simulink model "controladores_con_modulador"  (R2023b)
settings: Solver=FixedStepAuto  StartTime=0.0  StopTime=10.0  RelTol=1e-3
undefined symbols (not defined in the file): bh_eq_prima, DiscIntNeverNeededParam, i_h, Jh_eq_aux, Kd_h, Kd_t, Ki_h, Ki_t, Kp_h, Kp_t, r_hd, T_hm_max, T_s2, T_tm_max, tau_hm, tau_tm
settings Model: Creator=Ferran  LastModifiedBy=Ferran

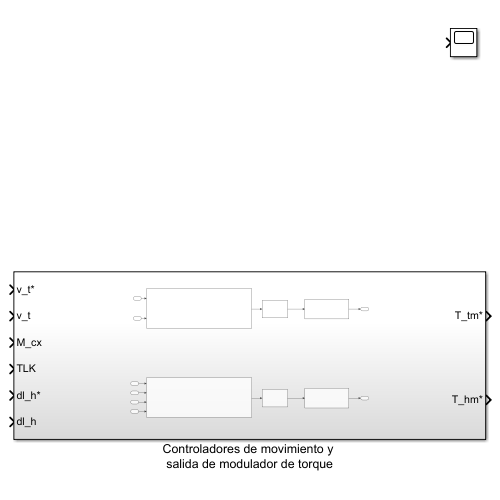
[thumbnail: Simulink's stored preview of the top-level diagram]
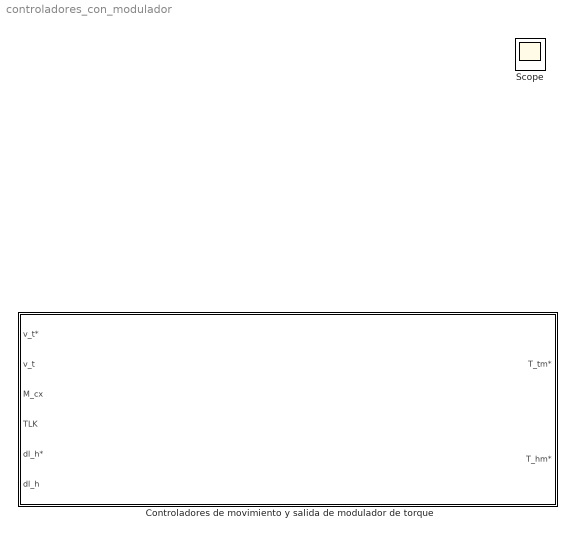
== system controladores_con_modulador ==
  Controladores de movimiento y salida de modulador de torque : Subsystem
  Scope : Scope

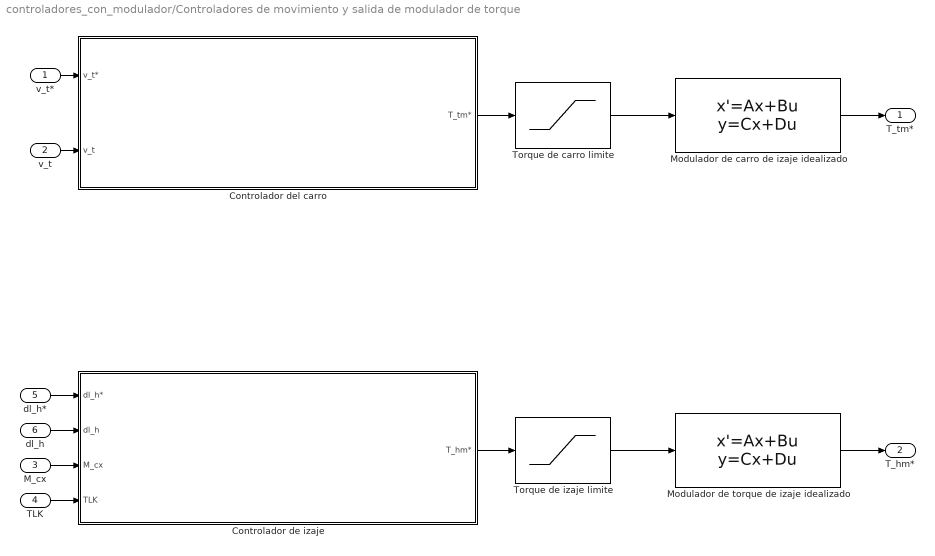
== system controladores_con_modulador/Controladores de movimiento y salida de modulador de torque ==
  v_t* : Inport
  v_t : Inport  Port=2
  M_cx : Inport  Port=3
  TLK : Inport  Port=4
  dl_h* : Inport  Port=5
  dl_h : Inport  Port=6
  Controlador de izaje : Subsystem
  Controlador del carro : Subsystem
  Modulador de carro de izaje idealizado : StateSpace  A=-1/tau_tm  B=1/tau_tm  D=0  InitialCondition=0
  Modulador de torque de izaje idealizado : StateSpace  A=-1/tau_hm  B=1/tau_hm  D=0  InitialCondition=0
  Torque de carro limite : Saturate  UpperLimit=T_tm_max  LowerLimit=-T_tm_max
  Torque de izaje limite : Saturate  UpperLimit=T_hm_max  LowerLimit=-T_hm_max
  T_tm* : Outport
  T_hm* : Outport  Port=2
  wires:
  dl_h*/1 -> Controlador de izaje/1(dl_h*)
  v_t/1 -> Controlador del carro/2(v_t)
  v_t*/1 -> Controlador del carro/1(v_t*)
  Controlador de izaje/1(T_hm*) -> Torque de izaje limite/1
  Controlador del carro/1(T_tm*) -> Torque de carro limite/1
  TLK/1 -> Controlador de izaje/4(TLK)
  dl_h/1 -> Controlador de izaje/2(dl_h)
  M_cx/1 -> Controlador de izaje/3(M_cx)
  Torque de izaje limite/1 -> Modulador de torque de izaje idealizado/1
  Torque de carro limite/1 -> Modulador de carro de izaje idealizado/1
  Modulador de carro de izaje idealizado/1 -> T_tm*/1
  Modulador de torque de izaje idealizado/1 -> T_hm*/1

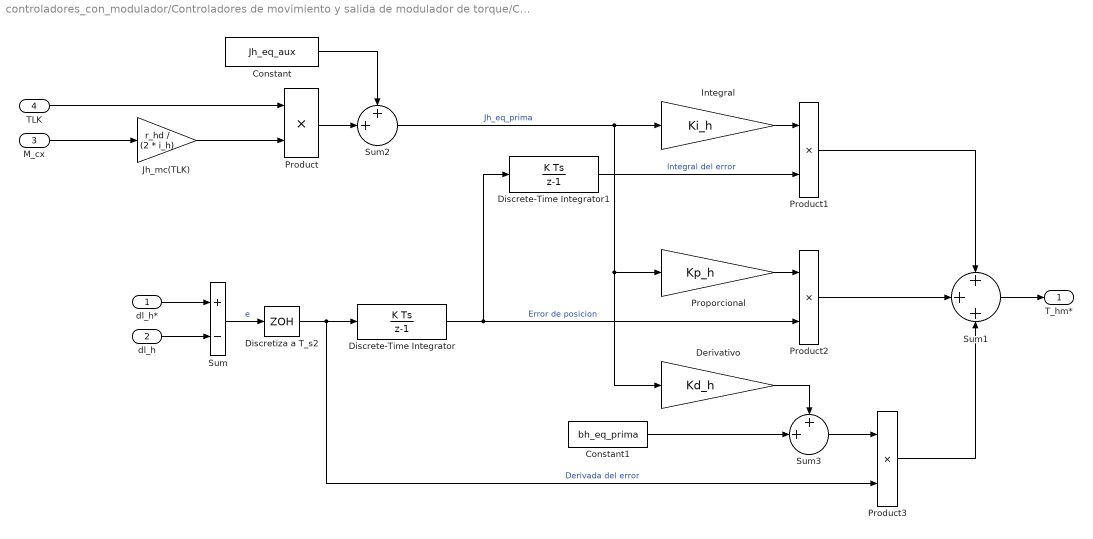
== system controladores_con_modulador/Controladores de movimiento y salida de modulador de torque/Controlador de izaje ==
  dl_h* : Inport
  dl_h : Inport  Port=2
  M_cx : Inport  Port=3
  TLK : Inport  Port=4
  Constant : Constant  Value=Jh_eq_aux
  Constant1 : Constant  Value=bh_eq_prima
  Derivativo : Gain  Gain=Kd_h
  Discrete-Time Integrator : DiscreteIntegrator  SampleTime=T_s2  ICPrevOutput=DiscIntNeverNeededParam  ICPrevScaledInput=DiscIntNeverNeededParam
  Discrete-Time Integrator1 : DiscreteIntegrator  SampleTime=T_s2  ICPrevOutput=DiscIntNeverNeededParam  ICPrevScaledInput=DiscIntNeverNeededParam
  Discretiza a T_s2 : ZeroOrderHold  SampleTime=T_s2
  Integral : Gain  Gain=Ki_h
  Jh_mc(TLK) : Gain  Gain=r_hd / (2 * i_h)
  Product{,1..3} (4 alike) : Product
  Proporcional : Gain  Gain=Kp_h
  Sum : Sum  Inputs=+-
  Sum1 : Sum  Inputs=+++
  Sum2 : Sum  Inputs=++|
  Sum3 : Sum  Inputs=++|
  T_hm* : Outport
  wires:
  dl_h*/1 -> Sum/1
  Product1/1 -> Sum1/1
  Discretiza a T_s2/1 -> Discrete-Time Integrator/1, Product3/2  "Derivada del error"
  dl_h/1 -> Sum/2
  Product3/1 -> Sum1/3
  Sum1/1 -> T_hm*/1
  Sum/1 -> Discretiza a T_s2/1  "e"
  Discrete-Time Integrator1/1 -> Product1/2  "Integral del error"
  M_cx/1 -> Jh_mc(TLK)/1
  Jh_mc(TLK)/1 -> Product/2
  TLK/1 -> Product/1
  Product/1 -> Sum2/2
  Constant/1 -> Sum2/1
  Sum2/1 -> Derivativo/1, Proporcional/1, Integral/1  "Jh_eq_prima"
  Integral/1 -> Product1/1
  Proporcional/1 -> Product2/1
  Discrete-Time Integrator/1 -> Product2/2, Discrete-Time Integrator1/1  "Error de posicion"
  Product2/1 -> Sum1/2
  Constant1/1 -> Sum3/2
  Derivativo/1 -> Sum3/1
  Sum3/1 -> Product3/1

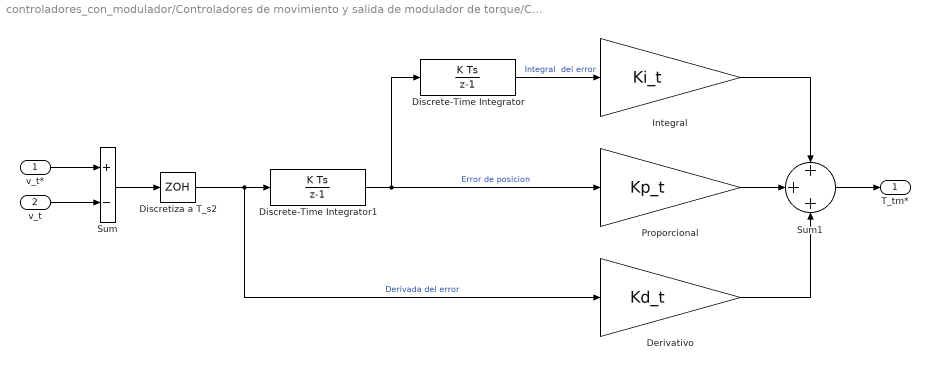
== system controladores_con_modulador/Controladores de movimiento y salida de modulador de torque/Controlador del carro ==
  v_t* : Inport
  v_t : Inport  Port=2
  Derivativo : Gain  Gain=Kd_t
  Discrete-Time Integrator : DiscreteIntegrator  SampleTime=T_s2  ICPrevOutput=DiscIntNeverNeededParam  ICPrevScaledInput=DiscIntNeverNeededParam
  Discrete-Time Integrator1 : DiscreteIntegrator  SampleTime=T_s2  ICPrevOutput=DiscIntNeverNeededParam  ICPrevScaledInput=DiscIntNeverNeededParam
  Discretiza a T_s2 : ZeroOrderHold  SampleTime=T_s2
  Integral : Gain  Gain=Ki_t
  Proporcional : Gain  Gain=Kp_t
  Sum : Sum  Inputs=+-
  Sum1 : Sum  Inputs=+++
  T_tm* : Outport
  wires:
  Discrete-Time Integrator1/1 -> Proporcional/1, Discrete-Time Integrator/1  "Error de posicion"
  v_t/1 -> Sum/2
  Discretiza a T_s2/1 -> Discrete-Time Integrator1/1, Derivativo/1  "Derivada del error"
  Sum/1 -> Discretiza a T_s2/1
  Derivativo/1 -> Sum1/3
  Integral/1 -> Sum1/1
  Sum1/1 -> T_tm*/1
  Discrete-Time Integrator/1 -> Integral/1  "Integral  del error"
  v_t*/1 -> Sum/1
  Proporcional/1 -> Sum1/2
